simulink library "ss_angles_2_vec"  (R2016b)
settings: Solver=VariableStepAuto  StartTime=0.0  StopTime=10.0  RelTol=1e-3
settings Model: Creator=taylorreynolds  LastModifiedBy=taylorreynolds

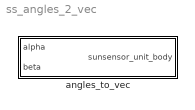
== system ss_angles_2_vec ==
  angles_to_vec : Subsystem

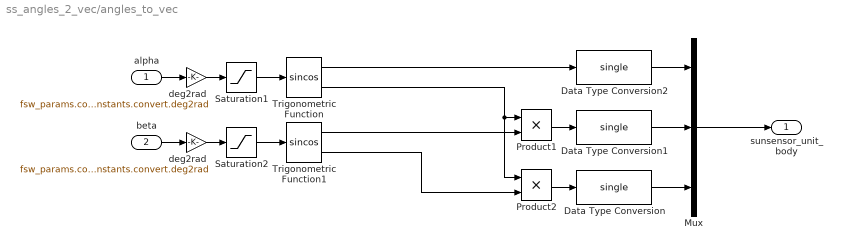
== system ss_angles_2_vec/angles_to_vec ==
  alpha : Inport
  beta : Inport  Port=2
  Data Type Conversion : DataTypeConversion  OutDataTypeStr=single
  Data Type Conversion1 : DataTypeConversion  OutDataTypeStr=single
  Data Type Conversion2 : DataTypeConversion  OutDataTypeStr=single
  Mux : Mux  Inputs=3
  Product1 : Product
  Product2 : Product
  Saturation1 : Saturate  UpperLimit=pi/2  LowerLimit=-pi/2
  Saturation2 : Saturate  UpperLimit=pi/2  LowerLimit=-pi/2
  Trigonometric Function : Trigonometry  Operator=sincos  OutputSignalType=real
  Trigonometric Function1 : Trigonometry  Operator=sincos  OutputSignalType=real
  deg2rad : Gain  Gain=fsw_params.constants.convert.deg2rad
  "deg2rad " : Gain  Gain=fsw_params.constants.convert.deg2rad
  sunsensor_unit_body : Outport
  wires:
  Data Type Conversion2/1 -> Mux/1
  Data Type Conversion1/1 -> Mux/2
  Data Type Conversion/1 -> Mux/3
  "deg2rad "/1 -> Saturation2/1
  deg2rad/1 -> Saturation1/1
  Mux/1 -> sunsensor_unit_body/1
  Product2/1 -> Data Type Conversion/1
  beta/1 -> "deg2rad "/1
  alpha/1 -> deg2rad/1
  Saturation1/1 -> Trigonometric Function/1
  Saturation2/1 -> Trigonometric Function1/1
  Trigonometric Function/1 -> Data Type Conversion2/1
  Product1/1 -> Data Type Conversion1/1
  Trigonometric Function1/1 -> Product1/2
  Trigonometric Function/2 -> Product2/1, Product1/1
  Trigonometric Function1/2 -> Product2/2
